simulink model "fixpt_dtc"  (R2015b)
settings: Solver=FixedStepDiscrete  StartTime=0.0  StopTime=0  FixedStep=1  RelTol=1e-3
settings Model: Creator=y_yama  LastModifiedBy=amatsumo
settings DataIOCC: SaveFormat=Array  SignalLoggingSaveFormat=ModelDataLogs  SaveOutput=off  SignalLogging=off  SaveTime=off
settings OptimizationCC: DefaultParameterBehavior=Inlined  InlineInvariantSignals=on  ExpressionDepthLimit=2147483647  ZeroExternalMemoryAtStartup=off  ZeroInternalMemoryAtStartup=off  InitFltsAndDblsToZero=on  NoFixptDivByZeroProtection=on  EfficientFloat2IntCast=on  OptimizeModelRefInitCode=on  LifeSpan=1
settings DebuggingCC: UnderspecifiedInitializationDetection=Classic  MergeDetectMultiDrivingBlocksExec=none  SolverPrmCheckMsg=warning  InheritedTsInSrcMsg=none  FcnCallInpInsideContextMsg=UseLocalSettings  StateNameClashWarn=warning
settings HardwareCC: ProdBitPerPointer=32  ProdLargestAtomicFloat=None  ProdWordSize=32  ProdHWDeviceType=Generic->32-bit Embedded Processor
settings RTWCC: SystemTargetFile=ert.tlc  GenCodeOnly=on  TemplateMakefile=ert_default_tmf  Description=Real-Time Workshop Embedded Coder (no auto configuration)  GenerateReport=on  IncludeHyperlinkInReport=on  LaunchReport=on
settings CodeAppCC: GenerateComments=off  IgnoreCustomStorageClasses=off  CustomSymbolStrGlobalVar=$N$M  CustomSymbolStrType=$N$R$M  SimulinkBlockComments=off  InternalIdentifier=Classic
settings ERTTargetCC: GenerateSampleERTMain=on  IncludeMdlTerminateFcn=off  SuppressErrorStatus=on  SupportAbsoluteTime=off  SupportNonFinite=off  SupportComplex=off  PurelyIntegerCode=on  InlinedParameterPlacement=NonHierarchical  ERTCustomFileTemplate=example_file_process.tlc
settings ConfigComp: CovModelRefEnable=Off  CovSFcnEnable=off

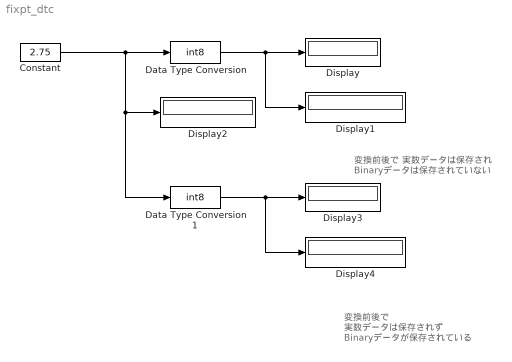
== system fixpt_dtc ==
  note: 変換前後で
      | 実数データは保存されず
      | Binaryデータが保存されている
  note: 変換前後で
      | 実数データは保存され
      | Binaryデータは保存されていない
  Constant : Constant  Value=2.75  OutDataTypeStr=fixdt(1,8,2)  SampleTime=-1
      settings: AttributesFormatString=DataType = %<OutDataTypeStr>
  Data Type Conversion : DataTypeConversion  OutDataTypeStr=int8  RndMeth=Nearest
      settings: AttributesFormatString=DataType = %<OutDataTypeStr>
  Data Type Conversion1 : DataTypeConversion  OutDataTypeStr=int8  ConvertRealWorld=Stored Integer (SI)  RndMeth=Nearest
      settings: AttributesFormatString=DataType = %<OutDataTypeStr>
  Display{,1..4} (5 alike) : Display
      Display settings: AttributesFormatString=Format = %<Format>
      Display1 settings: AttributesFormatString=Format = %<Format>  Format=binary (Stored Integer)
      Display2 settings: AttributesFormatString=Format = %<Format>  Format=binary (Stored Integer)
      Display3 settings: AttributesFormatString=Format = %<Format>
      Display4 settings: AttributesFormatString=Format = %<Format>  Format=binary (Stored Integer)
  wires:
  Constant/1 -> Data Type Conversion/1, Display2/1, Data Type Conversion1/1
  Data Type Conversion/1 -> Display/1, Display1/1
  Data Type Conversion1/1 -> Display3/1, Display4/1
